simulink model "Five_Phase_PWM"  (R2024a)
settings: Solver=FixedStepAuto  StartTime=0.0  StopTime=1  FixedStep=10e-6  RelTol=1e-3
libraries: simulink x1
settings Model: Creator=Ketan  LastModifiedBy=Ketan

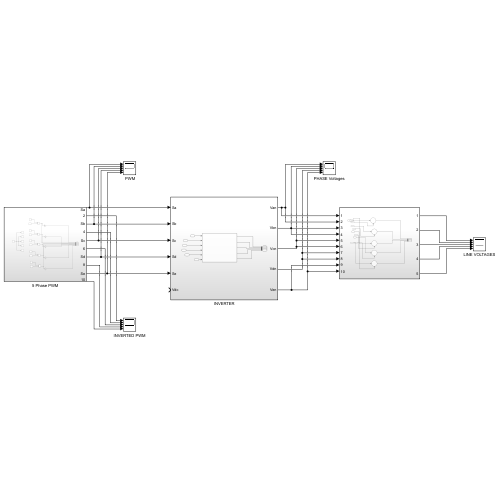
[thumbnail: Simulink's stored preview of the top-level diagram]
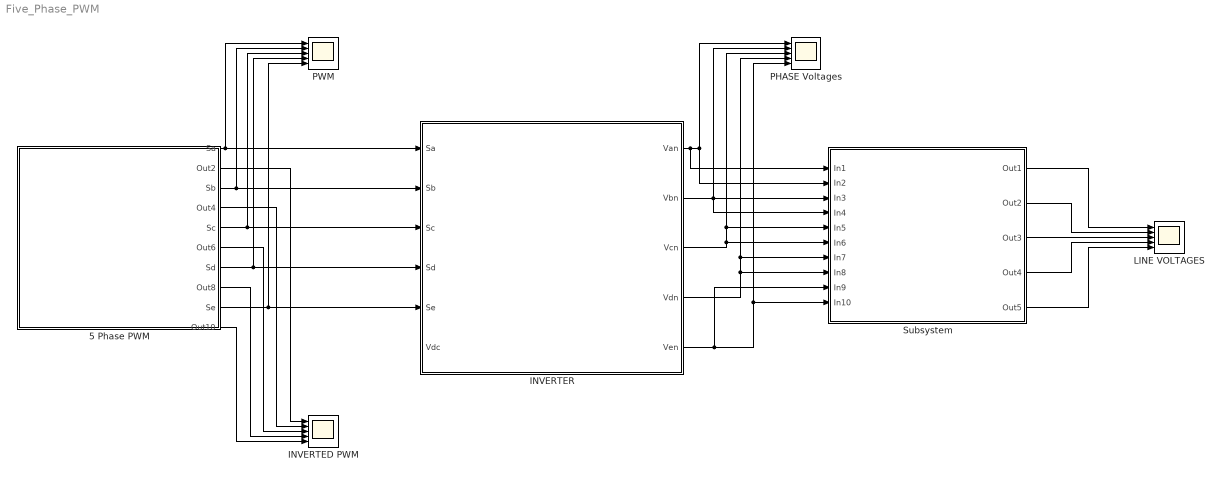
== system Five_Phase_PWM ==
  " PWM" : Scope  NumInputPorts=5
  5 Phase PWM : Subsystem
  INVERTED PWM : Scope  NumInputPorts=5
  INVERTER : Subsystem
  LINE VOLTAGES : Scope  NumInputPorts=5
  PHASE Voltages : Scope  NumInputPorts=5
  Subsystem : Subsystem
  wires:
  5 Phase PWM/1(Sa) -> " PWM"/1, INVERTER/1(Sa)
  5 Phase PWM/2(Out2) -> INVERTED PWM/1
  5 Phase PWM/3(Sb) -> " PWM"/2, INVERTER/2(Sb)
  5 Phase PWM/4(Out4) -> INVERTED PWM/2
  5 Phase PWM/5(Sc) -> " PWM"/3, INVERTER/3(Sc)
  5 Phase PWM/6(Out6) -> INVERTED PWM/3
  5 Phase PWM/7(Sd) -> " PWM"/4, INVERTER/4(Sd)
  5 Phase PWM/8(Out8) -> INVERTED PWM/4
  5 Phase PWM/9(Se) -> " PWM"/5, INVERTER/5(Se)
  5 Phase PWM/10(Out10) -> INVERTED PWM/5
  INVERTER/1(Van) -> Subsystem/1(In1), Subsystem/2(In2), PHASE Voltages/1
  INVERTER/2(Vbn) -> PHASE Voltages/2, Subsystem/3(In3), Subsystem/4(In4)
  INVERTER/3(Vcn) -> PHASE Voltages/3, Subsystem/5(In5), Subsystem/6(In6)
  INVERTER/4(Vdn) -> PHASE Voltages/4, Subsystem/7(In7), Subsystem/8(In8)
  INVERTER/5(Ven) -> Subsystem/9(In9), PHASE Voltages/5, Subsystem/10(In10)
  Subsystem/1(Out1) -> LINE VOLTAGES/1
  Subsystem/2(Out2) -> LINE VOLTAGES/2
  Subsystem/3(Out3) -> LINE VOLTAGES/3
  Subsystem/4(Out4) -> LINE VOLTAGES/4
  Subsystem/5(Out5) -> LINE VOLTAGES/5

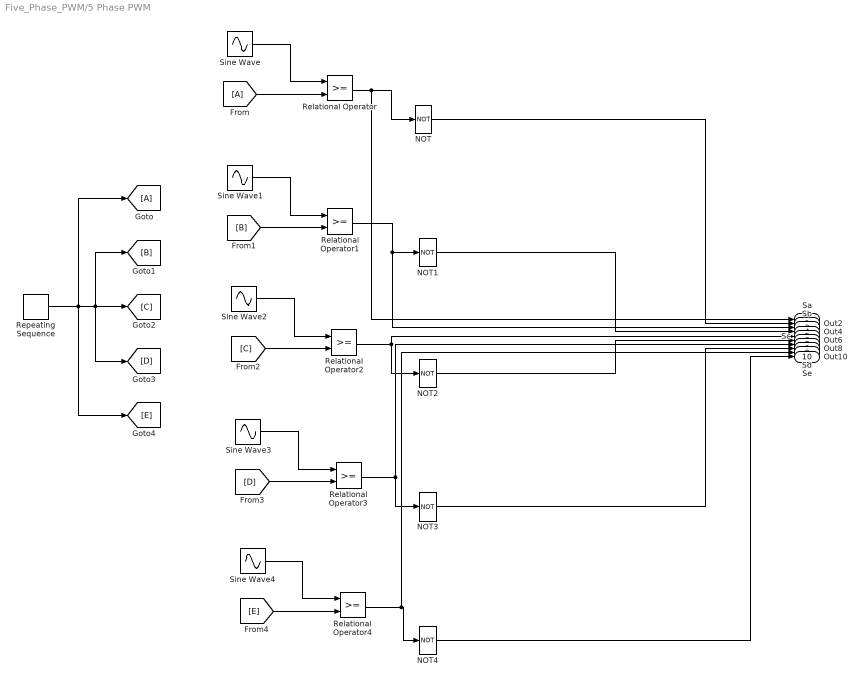
== system Five_Phase_PWM/5 Phase PWM ==
  From : From
  Goto : Goto
  NOT{,1..4} (5 alike) : Logic  Operator=NOT  IconShape=distinctive  AllPortsSameDT=off  OutDataTypeStr=boolean
  Relational Operator{,1..4} (5 alike) : RelationalOperator  OutDataTypeStr=boolean  RndMeth=Simplest  InputSameDT=off
  Repeating Sequence : simulink/Sources/Repeating Sequence  rep_seq_t=[0 0.25 0.5 0.75 1]*(1/5000)  rep_seq_y=[0 1 0 -1 0]
  Sine Wave : Sin  Amplitude=0.9  Frequency=2*pi*50  SampleTime=0
  Sine Wave1 : Sin  Amplitude=0.9  Frequency=2*pi*50  Phase=(2*pi)/5  SampleTime=0
  Sine Wave2 : Sin  Amplitude=0.9  Frequency=2*pi*50  Phase=(4*pi)/5  SampleTime=0
  Sine Wave3 : Sin  Amplitude=0.9  Frequency=2*pi*50  Phase=(6*pi)/5  SampleTime=0
  Sine Wave4 : Sin  Amplitude=0.9  Frequency=2*pi*50  Phase=(8*pi)/5  SampleTime=0
  Sa : Outport
  Out2 : Outport  Port=2
  Sb : Outport  Port=3
  Out4 : Outport  Port=4
  Sc : Outport  Port=5
  Out6 : Outport  Port=6
  Sd : Outport  Port=7
  Out8 : Outport  Port=8
  Se : Outport  Port=9
  Out10 : Outport  Port=10
  wires:
  Sine Wave1/1 -> Relational Operator1/1
  Sine Wave/1 -> Relational Operator/1
  Repeating Sequence/1 -> [E], Goto/1, [D], [B], [C]
  Relational Operator4/1 -> Se/1, NOT4/1
  Sine Wave2/1 -> Relational Operator2/1
  [E] -> Relational Operator4/2
  Sine Wave3/1 -> Relational Operator3/1
  Relational Operator1/1 -> Sb/1, NOT1/1
  [D] -> Relational Operator3/2
  Relational Operator3/1 -> Sd/1, NOT3/1
  Relational Operator2/1 -> Sc/1, NOT2/1
  Sine Wave4/1 -> Relational Operator4/1
  [B] -> Relational Operator1/2
  Relational Operator/1 -> Sa/1, NOT/1
  [C] -> Relational Operator2/2
  From/1 -> Relational Operator/2
  NOT/1 -> Out2/1
  NOT2/1 -> Out6/1
  NOT3/1 -> Out8/1
  NOT1/1 -> Out4/1
  NOT4/1 -> Out10/1

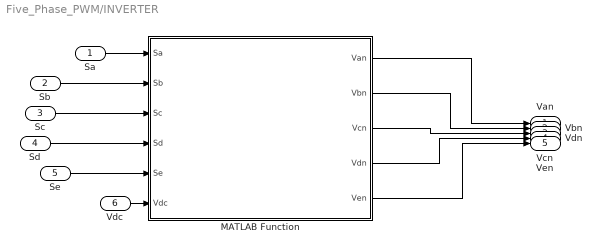
== system Five_Phase_PWM/INVERTER ==
  Sa : Inport
  Sb : Inport  Port=2
  Sc : Inport  Port=3
  Sd : Inport  Port=4
  Se : Inport  Port=5
  Vdc : Inport  Port=6
  MATLAB Function : MATLAB Function  TreatAsAtomicUnit=on
  Van : Outport
  Vbn : Outport  Port=2
  Vcn : Outport  Port=3
  Vdn : Outport  Port=4
  Ven : Outport  Port=5
  wires:
  Sa/1 -> MATLAB Function/1(Sa)
  Sc/1 -> MATLAB Function/3(Sc)
  MATLAB Function/2(Vbn) -> Vbn/1
  Sb/1 -> MATLAB Function/2(Sb)
  MATLAB Function/1(Van) -> Van/1
  MATLAB Function/3(Vcn) -> Vcn/1
  MATLAB Function/4(Vdn) -> Vdn/1
  MATLAB Function/5(Ven) -> Ven/1
  Vdc/1 -> MATLAB Function/6(Vdc)
  Se/1 -> MATLAB Function/5(Se)
  Sd/1 -> MATLAB Function/4(Sd)

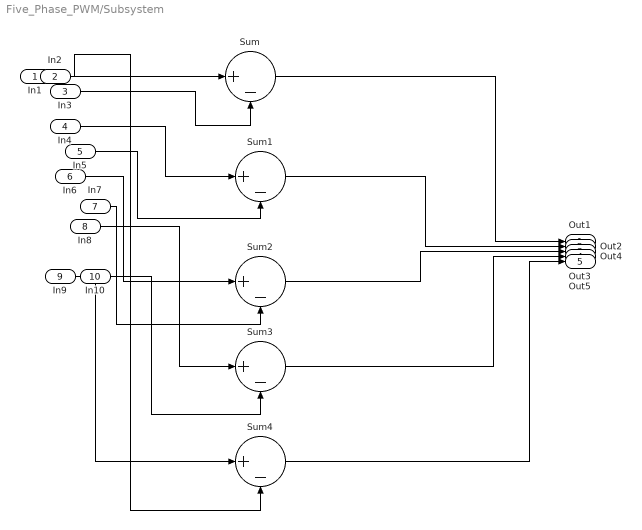
== system Five_Phase_PWM/Subsystem ==
  In1 : Inport
  In2 : Inport  Port=2
  In3 : Inport  Port=3
  In4 : Inport  Port=4
  In5 : Inport  Port=5
  In6 : Inport  Port=6
  In7 : Inport  Port=7
  In8 : Inport  Port=8
  In9 : Inport  Port=9
  In10 : Inport  Port=10
  Sum{,1..4} (5 alike) : Sum  Inputs=|+-
  Out1 : Outport
  Out2 : Outport  Port=2
  Out3 : Outport  Port=3
  Out4 : Outport  Port=4
  Out5 : Outport  Port=5
  wires:
  In10/1 -> Sum3/2
  In5/1 -> Sum1/2
  Sum4/1 -> Out5/1
  Sum/1 -> Out1/1
  In3/1 -> Sum/2
  In2/1 -> Sum/1
  In7/1 -> Sum2/2
  In1/1 -> Sum4/2
  In4/1 -> Sum1/1
  Sum3/1 -> Out4/1
  In8/1 -> Sum3/1
  In6/1 -> Sum2/1
  Sum2/1 -> Out3/1
  In9/1 -> Sum4/1
  Sum1/1 -> Out2/1

== matlab function Five_Phase_PWM/INVERTER/MATLAB Function ==
  data: Sa input; Van output; Sb input; Sc input; Sd input; Se input; Vdc input; Vbn output; Vcn output; Vdn output; Ven output
function [Van,Vbn,Vcn,Vdn,Ven]= fcn(Sa,Sb,Sc,Sd,Se,Vdc)
Vdc=100;
Van=(Vdc/2)*[(4*Sa)-Sb-Sc-Sd-Se];
Vbn=(Vdc/2)*[-Sa+(4*Sb)-Sc-Sd-Se];
Vcn=(Vdc/2)*[-Sa-Sb+(4*Sc)-Sd-Se];
Vdn=(Vdc/2)*[-Sa-Sb-Sc+(4*Sd)-Se];
Ven=(Vdc/2)*[-Sa-Sb-Sc-Sd+(4*Se)];
end
